simulink model "modeloSimulink"  (R2020a)
settings: Solver=VariableStepAuto  StartTime=t_initial  StopTime=t_final-h  FixedStep=h  RelTol=1e-3
undefined symbols (not defined in the file): A, B, C, D, h, x
settings Model: Creator=daniel  LastModifiedBy=daniel

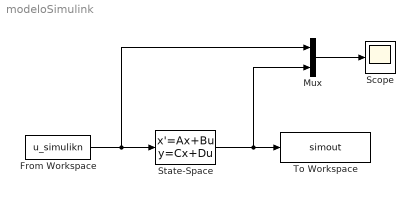
== system modeloSimulink ==
  From Workspace : FromWorkspace  VariableName=u_simulikn  SampleTime=h
  Mux : Mux  Inputs=2
  Scope : Scope
  State-Space : StateSpace  A=A  B=B  C=C  D=D  InitialCondition=x(:,1)
  To Workspace : ToWorkspace  VariableName=simout  SampleTime=-1
      settings: Save2DSignal=2-D array (concatenate along first dimension)
  wires:
  State-Space/1 -> Mux/2, To Workspace/1
  From Workspace/1 -> Mux/1, State-Space/1
  Mux/1 -> Scope/1
